simulink model "GalvoModel_servolike_v2"  (R2013a)
settings: Solver=ode45  StartTime=0.0  StopTime=10.0  RelTol=1e-3
undefined symbols (not defined in the file or in its folder): BEM, CL, CR, FR, KTR, RIN, TRC
settings Model: Creator=mainster  LastModifiedBy=mainster
settings DebuggingCC: SolverPrmCheckMsg=none

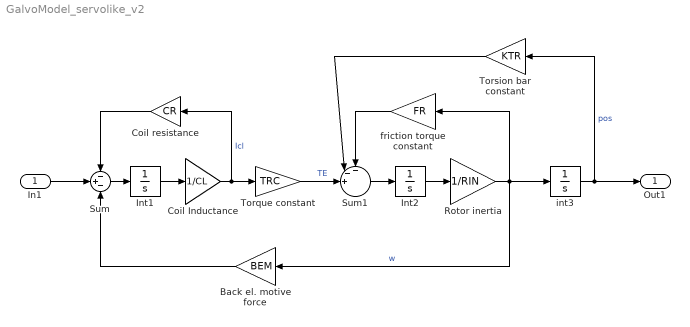
== system GalvoModel_servolike_v2 ==
  In1 : Inport
  Back el. motive force : Gain  Gain=BEM
  Coil Inductance : Gain  Gain=1/CL
  Coil resistance : Gain  Gain=CR
  Int1 : Integrator
  Int2 : Integrator
  Rotor inertia : Gain  Gain=1/RIN
  Sum : Sum  Inputs=-+-
  Sum1 : Sum  Inputs=--+||
  Torque constant : Gain  Gain=TRC
  Torsion bar constant : Gain  Gain=KTR
  friction torque constant : Gain  Gain=FR
  int3 : Integrator
  Out1 : Outport
  wires:
  Sum/1 -> Int1/1
  Rotor inertia/1 -> Back el. motive force/1, int3/1, friction torque constant/1  "w"
  int3/1 -> Torsion bar constant/1, Out1/1  "pos"
  Int1/1 -> Coil Inductance/1
  Coil Inductance/1 -> Coil resistance/1, Torque constant/1  "Icl"
  Coil resistance/1 -> Sum/1
  Back el. motive force/1 -> Sum/3
  Int2/1 -> Rotor inertia/1
  friction torque constant/1 -> Sum1/1
  Torsion bar constant/1 -> Sum1/2
  Torque constant/1 -> Sum1/3  "TE"
  Sum1/1 -> Int2/1
  In1/1 -> Sum/2
